simulink model "SA_ACC_UIO_sim"  (R2020b)
settings: Solver=FixedStepDiscrete  StartTime=0.0  StopTime=20  FixedStep=0.01  RelTol=1e-3
PreLoadFcn:
  | li = 5;
  | Li = 7.3;
  | h = 0.5;
  | k1 = -0.8;
  | k2 = 2.5;
  | Ts = 0.01;
values from neighbouring files (symbols this model uses):
  Ad = (eye(length(Ac))+Ts*Ac)    [SA_ACC_UIO.m]    (also in init_uio.m; init_uio_new.m)
  Bd = Ts*Bc    [SA_ACC_UIO.m]    (also in init_uio.m; init_uio_new.m)
  Cd = Cc    [SA_ACC_UIO.m]    (also in init_uio.m; init_uio_new.m)
  deltad = Ts*deltac    [SA_ACC_UIO.m]    (also in init_uio.m; init_uio_new.m)
  Fd = Ts*Fc    [SA_ACC_UIO.m]    (also in init_uio.m; init_uio_new.m)
  G = Pz*Fe    [SA_ACC_UIO.m]    (also in init_uio.m; init_uio_new.m)
  L = K+N*Qz    [SA_ACC_UIO.m]    (also in init_uio.m; init_uio_new.m)
  M = Pz*Be    [SA_ACC_UIO.m]    (also in init_uio.m; init_uio_new.m)
  N = Az-K*Ce    [SA_ACC_UIO.m]    (also in init_uio.m; init_uio_new.m)
  Pz = g_invEC(1:4,1:3)    [SA_ACC_UIO.m]    (also in init_uio.m; init_uio_new.m)
  Qz = g_invEC(:,4:5)    [SA_ACC_UIO.m]    (also in init_uio.m; init_uio_new.m)
  Wd = Ts*Wc    [SA_ACC_UIO.m]    (also in init_uio.m; init_uio_new.m)
libraries: commrandsrc3 x1
settings Model: Creator=oussa  LastModifiedBy=KSL
settings DataIOCC: ReturnWorkspaceOutputs=off
settings DebuggingCC: ArithmeticOperatorsInVariantConditions=warning
settings SFSimCC: SimUseLocalCustomCode=off  CustomCodeUndefinedFunction=UseInterfaceOnly
settings RTWCC: RTWUseLocalCustomCode=off

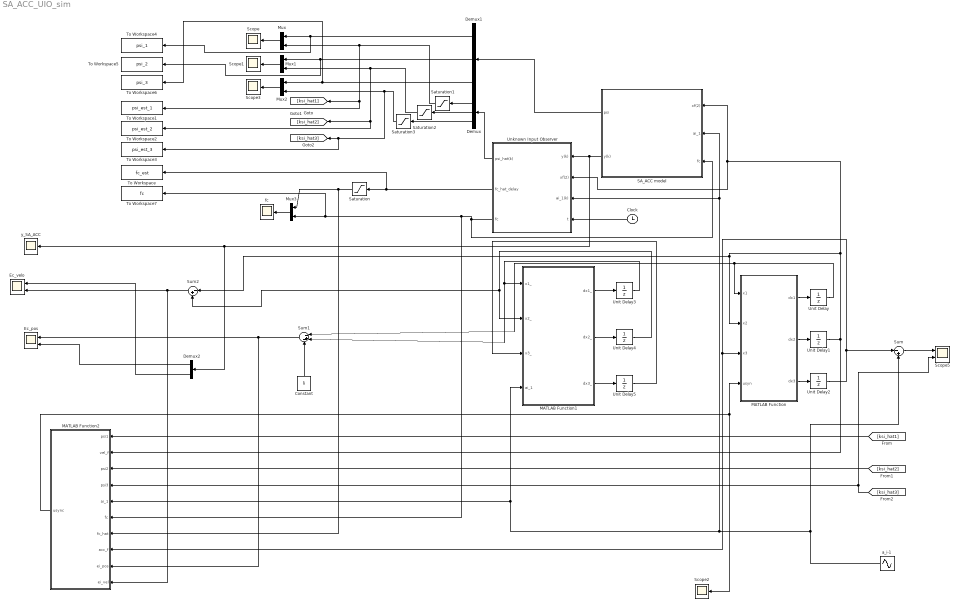
== system SA_ACC_UIO_sim ==
  Clock : Clock
  Constant : Constant  Value=li
  Demux : Demux  Outputs=3
  Demux1 : Demux  Outputs=3
  Demux2 : Demux  Outputs=2
  Ec_pos : Scope  NumInputPorts=2
  Ec_velo : Scope  NumInputPorts=2
  MATLAB Function : MATLAB Function  TreatAsAtomicUnit=on
  MATLAB Function1 : MATLAB Function  TreatAsAtomicUnit=on
  MATLAB Function2 : MATLAB Function  TreatAsAtomicUnit=on
  Mux{,1..3} (4 alike) : Mux  Inputs=2
  SA_ACC model : Subsystem
  Saturation : Saturate  UpperLimit=15  LowerLimit=-10
  Saturation1 : Saturate  UpperLimit=100  LowerLimit=-20
  Saturation2 : Saturate  UpperLimit=20  LowerLimit=-20
  Saturation3 : Saturate  UpperLimit=20  LowerLimit=-20
  Scope{,1..3} (4 alike) : Scope
  Scope5 : Scope  NumInputPorts=2
  Sum : Sum  Inputs=|-+
  Sum1 : Sum  Inputs=|-+-
  Sum2 : Sum  Inputs=|-+
  To Workspace : ToWorkspace  VariableName=fc_est  SaveFormat=Timeseries  SampleTime=-1
  To Workspace1 : ToWorkspace  VariableName=psi_est_1  SaveFormat=Timeseries  SampleTime=-1
  To Workspace2 : ToWorkspace  VariableName=psi_est_2  SaveFormat=Timeseries  SampleTime=-1
  To Workspace3 : ToWorkspace  VariableName=psi_est_3  SaveFormat=Timeseries  SampleTime=-1
  To Workspace4 : ToWorkspace  VariableName=psi_1  SaveFormat=Timeseries  SampleTime=-1
  To Workspace5 : ToWorkspace  VariableName=psi_2  SaveFormat=Timeseries  SampleTime=-1
  To Workspace6 : ToWorkspace  VariableName=psi_3  SaveFormat=Timeseries  SampleTime=-1
  To Workspace7 : ToWorkspace  VariableName=fc  SaveFormat=Timeseries  SampleTime=-1
  Unit Delay{,1..2,5} (4 alike) : UnitDelay  SampleTime=-1  HasFrameUpgradeWarning=on
  Unit Delay3 : UnitDelay  InitialCondition=10  SampleTime=-1  HasFrameUpgradeWarning=on
  Unit Delay4 : UnitDelay  InitialCondition=10  SampleTime=-1  HasFrameUpgradeWarning=on
  Unknown Input Observer : Subsystem
  a_i-1 : Sin  Amplitude=3  Frequency=2*pi/10  SampleTime=Ts
  fc : Scope
  y_SA_ACC : Scope
  wires:
  MATLAB Function/1(dx1) -> Unit Delay/1
  MATLAB Function/2(dx2) -> Unit Delay1/1
  MATLAB Function/3(dx3) -> Unit Delay2/1
  Unit Delay2/1 -> Sum/1, MATLAB Function/3(x3), MATLAB Function2/8(acc_f)
  MATLAB Function1/1(dx1_) -> Unit Delay3/1
  MATLAB Function1/2(dx2_) -> Unit Delay4/1
  MATLAB Function1/3(dx3_) -> Unit Delay5/1
  Unit Delay4/1 -> MATLAB Function1/2(x2_), Sum2/2
  Unit Delay5/1 -> MATLAB Function1/3(x3_)
  Unknown Input Observer/2(fc_hat_delay) -> To Workspace/1, Saturation/1
  Demux/1 -> Saturation1/1
  Demux/2 -> Saturation2/1
  Demux/3 -> Saturation3/1
  Unknown Input Observer/1(psi_hat(k)) -> Demux/1
  SA_ACC model/1(psi) -> Demux1/1
  Demux1/1 -> To Workspace4/1, Mux/1
  Demux1/2 -> To Workspace5/1, Mux1/1
  Saturation2/1 -> [ksi_hat2], To Workspace2/1, Mux1/2
  Mux1/1 -> Scope1/1
  Demux1/3 -> To Workspace6/1, Mux2/1
  Saturation3/1 -> To Workspace3/1, [ksi_hat3], Mux2/2
  Mux/1 -> Scope/1
  Mux2/1 -> Scope3/1
  Saturation/1 -> Mux3/1, MATLAB Function2/7(fc_hat)
  Mux3/1 -> fc/1
  MATLAB Function2/1(usync) -> Scope2/1, MATLAB Function/4(usyn)
  Unit Delay1/1 -> MATLAB Function2/2(vel_f), Unknown Input Observer/2(xf(2)), SA_ACC model/1(xf(2)), MATLAB Function/2(x2), Sum2/1
  a_i-1/1 -> Sum/2, SA_ACC model/2(ai_1), Unknown Input Observer/3(ai_1(k)), MATLAB Function1/4(ai_1), MATLAB Function2/5(ai_1)
  Unknown Input Observer/3(fc) -> SA_ACC model/3(fc), MATLAB Function2/6(fc), To Workspace7/1, Mux3/2
  [ksi_hat1] -> MATLAB Function2/1(psi1)
  Saturation1/1 -> To Workspace1/1, [ksi_hat1], Mux/2
  [ksi_hat3] -> MATLAB Function2/4(psi3), Scope5/2
  [ksi_hat2] -> MATLAB Function2/3(psi2)
  Sum/1 -> Scope5/1
  Clock/1 -> Unknown Input Observer/4(t)
  SA_ACC model/2(y(k)) -> y_SA_ACC/1, Demux2/1, Unknown Input Observer/1(y(k))
  Unit Delay/1 -> Sum1/1, MATLAB Function/1(x1)
  Unit Delay3/1 -> MATLAB Function1/1(x1_), Sum1/2
  Demux2/1 -> Ec_pos/2
  Demux2/2 -> Ec_velo/1
  Constant/1 -> Sum1/3
  Sum1/1 -> MATLAB Function2/9(ei_pos), Ec_pos/1
  Sum2/1 -> MATLAB Function2/10(ei_vel), Ec_velo/2

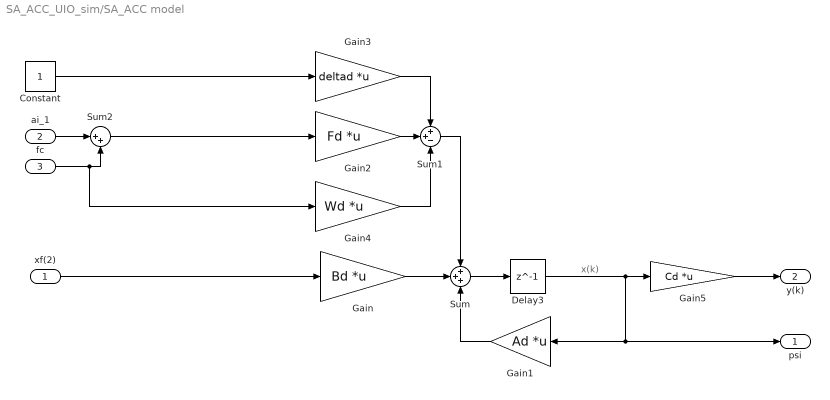
== system SA_ACC_UIO_sim/SA_ACC model ==
  note: x(k)
  xf(2) : Inport
  ai_1 : Inport  Port=2
  fc : Inport  Port=3
  Constant : Constant
  Delay3 : Delay  DelayLength=1  InitialCondition=[5;10;0]
  Gain : Gain  Gain=Bd  Multiplication=Matrix(K*u) (u vector)
  Gain1 : Gain  Gain=Ad  Multiplication=Matrix(K*u) (u vector)
  Gain2 : Gain  Gain=Fd  Multiplication=Matrix(K*u) (u vector)
  Gain3 : Gain  Gain=deltad  Multiplication=Matrix(K*u) (u vector)
  Gain4 : Gain  Gain=Wd  Multiplication=Matrix(K*u) (u vector)
  Gain5 : Gain  Gain=Cd  Multiplication=Matrix(K*u) (u vector)
  Sum : Sum  Inputs=+++
  Sum1 : Sum  Inputs=++-
  Sum2 : Sum  Inputs=|++
  psi : Outport  VectorParamsAs1DForOutWhenUnconnected=off
  y(k) : Outport  Port=2  VectorParamsAs1DForOutWhenUnconnected=off
  wires:
  Sum/1 -> Delay3/1
  Delay3/1 -> Gain5/1, psi/1, Gain1/1
  xf(2)/1 -> Gain/1
  Gain5/1 -> y(k)/1
  Gain1/1 -> Sum/3
  Gain/1 -> Sum/2
  Gain2/1 -> Sum1/2
  Sum1/1 -> Sum/1
  Constant/1 -> Gain3/1
  Gain3/1 -> Sum1/1
  fc/1 -> Gain4/1, Sum2/2
  ai_1/1 -> Sum2/1
  Sum2/1 -> Gain2/1
  Gain4/1 -> Sum1/3

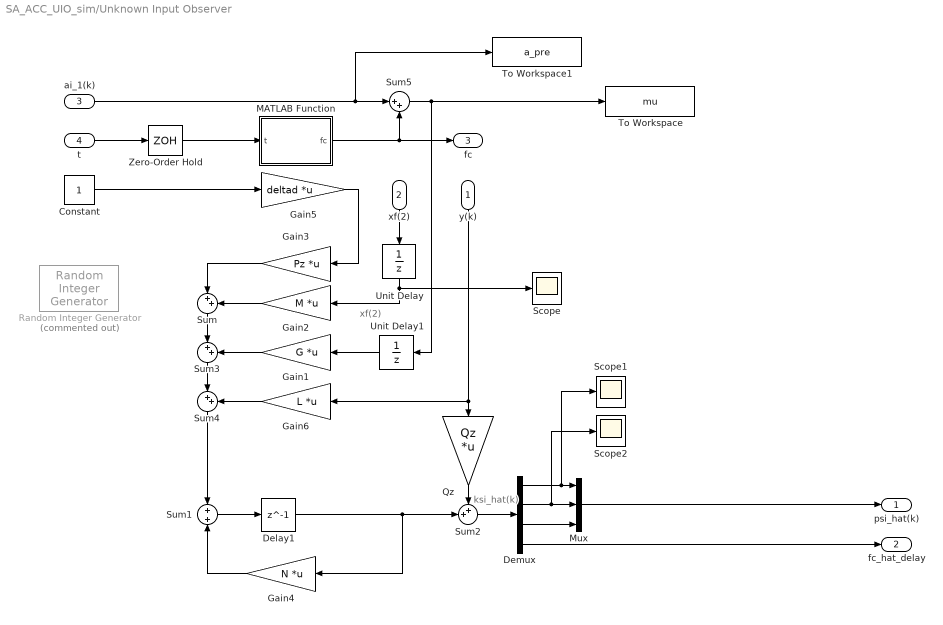
== system SA_ACC_UIO_sim/Unknown Input Observer ==
  note: xf(2)
  note: ksi_hat(k)
  y(k) : Inport
  xf(2) : Inport  Port=2
  ai_1(k) : Inport  Port=3
  t : Inport  Port=4
  Constant : Constant
  Delay1 : Delay  DelayLength=1  InitialCondition=[0;0;0;0]
  Demux : Demux
  Gain1 : Gain  Gain=G  Multiplication=Matrix(K*u) (u vector)
  Gain2 : Gain  Gain=M  Multiplication=Matrix(K*u) (u vector)
  Gain3 : Gain  Gain=Pz  Multiplication=Matrix(K*u) (u vector)
  Gain4 : Gain  Gain=N  Multiplication=Matrix(K*u) (u vector)
  Gain5 : Gain  Gain=deltad  Multiplication=Matrix(K*u) (u vector)
  Gain6 : Gain  Gain=L  Multiplication=Matrix(K*u) (u vector)
  MATLAB Function : MATLAB Function  TreatAsAtomicUnit=on
  Mux : Mux  Inputs=3
  Qz : Gain  Gain=Qz  Multiplication=Matrix(K*u) (u vector)
  Random Integer Generator : commrandsrc3/Random Integer Generator  Commented=on  SetSize=8  SeedSource=Auto  Seed=0  SampleTime=0.05  SamplesPerFrame=1  OutputDataType=double  SimulateUsing=Interpreted execution
  Scope : Scope
  Scope1 : Scope
  Scope2 : Scope
  Sum{,3..5} (4 alike) : Sum  Inputs=|++
  Sum1 : Sum
  Sum2 : Sum  Inputs=++|
  To Workspace : ToWorkspace  VariableName=mu  SaveFormat=Timeseries  SampleTime=-1
  To Workspace1 : ToWorkspace  VariableName=a_pre  SaveFormat=Timeseries  SampleTime=-1
  Unit Delay : UnitDelay  SampleTime=-1  HasFrameUpgradeWarning=on
  Unit Delay1 : UnitDelay  SampleTime=-1  HasFrameUpgradeWarning=on
  Zero-Order Hold : ZeroOrderHold  SampleTime=-1
  psi_hat(k) : Outport  VectorParamsAs1DForOutWhenUnconnected=off
  fc_hat_delay : Outport  Port=2  VectorParamsAs1DForOutWhenUnconnected=off
  fc : Outport  Port=3  VectorParamsAs1DForOutWhenUnconnected=off
  wires:
  Qz/1 -> Sum2/1
  y(k)/1 -> Gain6/1, Qz/1
  Gain4/1 -> Sum1/2
  Delay1/1 -> Sum2/2, Gain4/1
  Sum1/1 -> Delay1/1
  Sum2/1 -> Demux/1
  Demux/1 -> Scope1/1, Mux/1
  Demux/2 -> Scope2/1, Mux/2
  Mux/1 -> psi_hat(k)/1
  Demux/4 -> fc_hat_delay/1
  Demux/3 -> Mux/3
  Sum5/1 -> Unit Delay1/1, To Workspace/1
  xf(2)/1 -> Unit Delay/1
  Gain5/1 -> Gain3/1
  Gain2/1 -> Sum/2
  Gain3/1 -> Sum/1
  Sum/1 -> Sum3/1
  Gain1/1 -> Sum3/2
  Gain6/1 -> Sum4/2
  Sum3/1 -> Sum4/1
  Sum4/1 -> Sum1/1
  Constant/1 -> Gain5/1
  ai_1(k)/1 -> To Workspace1/1, Sum5/1
  Unit Delay/1 -> Gain2/1, Scope/1
  Unit Delay1/1 -> Gain1/1
  t/1 -> Zero-Order Hold/1
  Zero-Order Hold/1 -> MATLAB Function/1(t)
  MATLAB Function/1(fc) -> fc/1, Sum5/2

== matlab function SA_ACC_UIO_sim/MATLAB Function1 ==
  data: x1_ input; dx1_ output; x2_ input; x3_ input; dx2_ output; dx3_ output; ai_1 input
function [dx1_,dx2_,dx3_] = preceeding(x1_,x2_,x3_,ai_1)


Ts = 1/100;

Ai_ = [1 Ts 0;
       0 1 0;
       0 0 1];



dx1_ = Ai_(1,:)*[x1_;x2_;x3_];
dx2_ = Ai_(2,:)*[x1_;x2_;x3_]+Ts*ai_1;
dx3_ = Ai_(3,:)*[x1_;x2_;x3_] ;

== matlab function SA_ACC_UIO_sim/MATLAB Function ==
  data: x1 input; dx1 output; x2 input; x3 input; dx2 output; dx3 output; usyn input
function [dx1,dx2,dx3] = following(x1,x2,x3,usyn)


Ts = 1/100;
tau = 0.4;

Ai = [1 Ts 0;0 1 Ts;0 0 1-Ts/tau];

% x = [x1;x2;x3];
dx1 = Ai(1,:)*[x1;x2;x3];
dx2 = Ai(2,:)*[x1;x2;x3];
dx3 = Ai(3,:)*[x1;x2;x3]+Ts/tau*usyn ;

% dx = Ai*x;
% dx1 = dx(1,:)
% dx2 = dx(2,:)
% dx3 = dx(3,:)*[x1;x2;x3]+Ts/tau*usyn;

== matlab function SA_ACC_UIO_sim/MATLAB Function2 ==
  data: psi1 input; vel_f input; psi2 input; psi3 input; usync output; ai_1 input; fc input; fc_hat input; acc_f input; ei_pos input; ei_vel input
 function usync = control(psi1,vel_f,psi2,psi3,ai_1,fc,fc_hat,acc_f,ei_pos,ei_vel)

persistent frame 

if isempty(frame)
    frame = 0;
end
Ts = 1/100;
tau = 0.4;


li = 5;
Li = 8;
h = 0.5;
k1 = -0.8;
k2 = 2.5;

a1 = h*k1*k2;
a2 = -k2;
b1 = -(k1+h*k1*k2);
k3 = (1-h*k1*k2);
b3 = k2/h;
c = -k2/h*(Li-li);

mu = (ai_1+fc);
usync = h*k1*k2*mu-(k1+h*k1*k2)*fc_hat-k2*vel_f-(k1+h*k1*k2)*(psi3)...
        +k3/h*(psi2)+k2/h*(psi1)-k2/h*(Li-li);
% usync = a1*ai_1+a2*x2+b1*(x3_-x3)+b2*(x2_-x2)+b3*(x1_-x1-li)+c;
% if (frame*Ts > 2 && abs(fc_hat) > 0)
%     usync = h*k1*k2*mu-(k1+h*k1*k2)*fc_hat-k2*x2-(k1+h*k1*k2)*(psi3)...
%         +k3/h*(psi2)+k2/h*(psi1)-k2/h*(Li-li);
% else
%     usync = -k1*mu+(k1+h*k1*k2)*acc_f ...
%                    -1/h*(1-h*k1*k2)*ei_vel-k2/h*ei_pos-k2*x2; % original
% end       
frame = frame + 1;

== matlab function SA_ACC_UIO_sim/Unknown Input Observer/MATLAB Function ==
  data: t input; fc output
function fc = attack(t)

% %% Case linear attaack
    if (t < 6)
        fc = 0;
    elseif (t >=6 && t<12)
        %%# print(time_eslap)
        fc = 2*(t - 4);
%     elseif (t>=9 && t<16)
%         fc = 5;
    else
        fc = 5;
    end
%     
%% Case linear attaack
%     fc = 5;
%% Case bla bla 
%     if t<4
%         fc = 0;
%     elseif t >=4 && t<8
%         fc = 10*sin(10*pi/2*t)*exp(-0.01*(t));
%     elseif t>=9 && t<16
%         fc =  3*exp(-2*sin(10*pi/2*t)*0.01*(t));
%     else
%         fc =  0;%3;
%         

%% Case random attack
    
%     if t<4
%         fc = 0;
%     elseif t >=4 && t<16
%         if (randsample(10,1) >= 8)
%             fc = -5 + (5+5)*rand();
%         else 
%             fc = 0;
%         end
%     else
%         fc =  0;%3
%     end
